simulink model "LoadPosition_simul"  (R2017a)
settings: Solver=FixedStepAuto  StartTime=0.0  StopTime=sim_time  FixedStep=delta  RelTol=1e-3
values from neighbouring files (symbols this model uses):
  A = [0.717 -1.367 -0.218 -0.867 -0.899 ... (first row only)    [LoadPosition_main.m]
  B = [0.083; 0.056; -0.056; 0.111; -0.056]    [LoadPosition_main.m]
  C = [0 1 1 0 0]    [LoadPosition_main.m]
  delta = 0.001    [LoadPosition_main.m]
  Dis_instant = 10    [LoadPosition_main.m]
  Dis_interval = 3    [LoadPosition_main.m]
  Dis_size = 5    [LoadPosition_main.m]
  K = place(A,B,poles)    [LoadPosition_main.m]
undefined symbols (not defined in the file or in its folder): A_, B_
settings Model: Creator=sihoon  LastModifiedBy=root

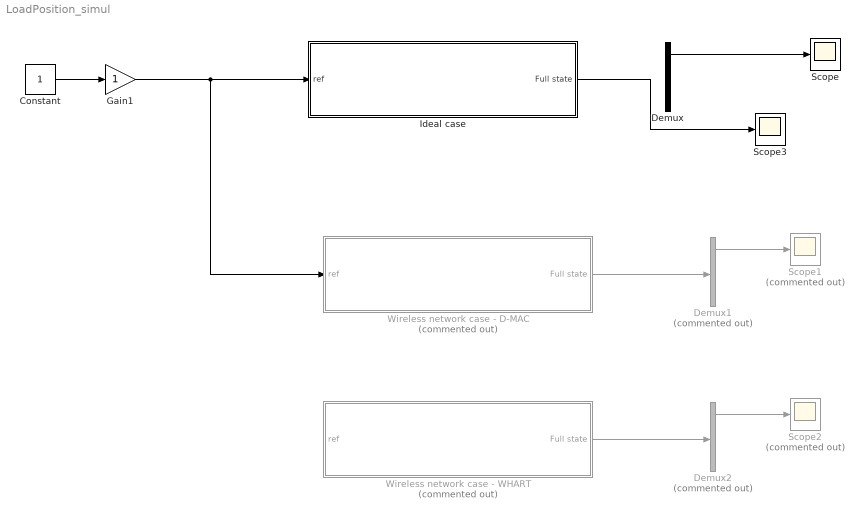
== system LoadPosition_simul ==
  Constant : Constant
  Demux : Demux
  Demux1 : Demux  Commented=on
  Demux2 : Demux  Commented=on
  Gain1 : Gain
  "Ideal case " : Subsystem
  Scope : Scope
  Scope1 : Scope  Commented=on
  Scope2 : Scope  Commented=on
  Scope3 : Scope
  Wireless network case - D-MAC : Subsystem  Commented=on
  Wireless network case - WHART : Subsystem  Commented=on
  wires:
  Constant/1 -> Gain1/1
  Demux/1 -> Scope/1
  "Ideal case "/1(Full state) -> Scope3/1
  Gain1/1 -> Wireless network case - D-MAC/1(ref), "Ideal case "/1(ref)
  Demux1/1 -> Scope1/1
  Wireless network case - D-MAC/1(Full state) -> Demux1/1
  Wireless network case - WHART/1(Full state) -> Demux2/1
  Demux2/1 -> Scope2/1

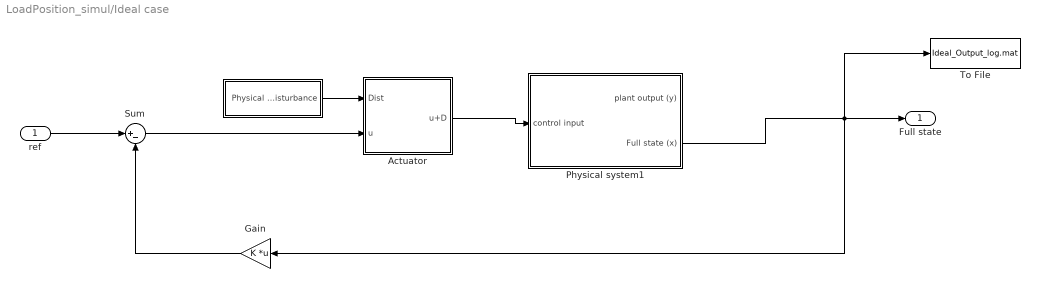
== system LoadPosition_simul/Ideal case  ==
  ref : Inport
  " " : Subsystem
  Actuator : Subsystem
  Gain : Gain  Gain=K  Multiplication=Matrix(K*u)
  Physical system1 : Subsystem
  Sum : Sum  Inputs=|+-
  To File : ToFile  Filename=Ideal_Output_log.mat  SaveFormat=Timeseries
  Full state : Outport
  wires:
  Physical system1/2(Full state (x)) -> Gain/1, Full state/1, To File/1
  Gain/1 -> Sum/2
  Sum/1 -> Actuator/2(u)
  ref/1 -> Sum/1
  " "/1(Physical Disturbance) -> Actuator/1(Dist)
  Actuator/1(u+D) -> Physical system1/1(control input)

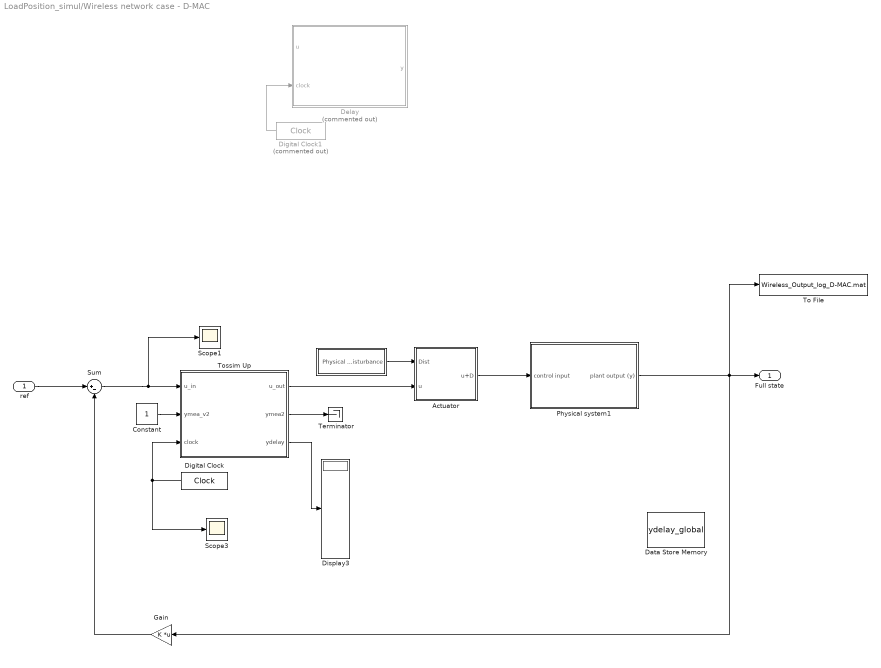
== system LoadPosition_simul/Wireless network case - D-MAC ==
  ref : Inport
  " " : Subsystem
  Actuator : Subsystem
  Constant : Constant
  Data Store Memory : DataStoreMemory  DataStoreName=ydelay_global  ReadBeforeWriteMsg=warning  WriteAfterWriteMsg=warning  WriteAfterReadMsg=warning  InitialValue=[1; 1; 1; 1; 1; 1; 1; 1; 1; 1; 1; 1; 1; 1; 1]  ShowAdditionalParam=off  OutDataTypeStr=uint32
  Delay : MATLAB Function  Commented=on  TreatAsAtomicUnit=on
  Digital Clock : DigitalClock  SampleTime=delta
  Digital Clock1 : DigitalClock  Commented=on  SampleTime=delta
  Display3 : Display
  Gain : Gain  Gain=K  Multiplication=Matrix(K*u)
  Physical system1 : Subsystem
  Scope1 : Scope
  Scope3 : Scope
  Sum : Sum  Inputs=|+-
  Terminator : Terminator
  To File : ToFile  Filename=Wireless_Output_log_D-MAC.mat  SaveFormat=Timeseries
  Tossim Up : MATLAB Function  TreatAsAtomicUnit=on
  Full state : Outport
  wires:
  Physical system1/1(plant output (y)) -> Gain/1, Full state/1, To File/1
  Gain/1 -> Sum/2
  ref/1 -> Sum/1
  Constant/1 -> Tossim Up/2(ymea_v2)
  Tossim Up/3(ydelay) -> Display3/1
  Digital Clock/1 -> Tossim Up/3(clock), Scope3/1
  Tossim Up/2(ymea2) -> Terminator/1
  Tossim Up/1(u_out) -> Actuator/2(u)
  Digital Clock1/1 -> Delay/2(clock)
  Sum/1 -> Tossim Up/1(u_in), Scope1/1
  " "/1(Physical Disturbance) -> Actuator/1(Dist)
  Actuator/1(u+D) -> Physical system1/1(control input)

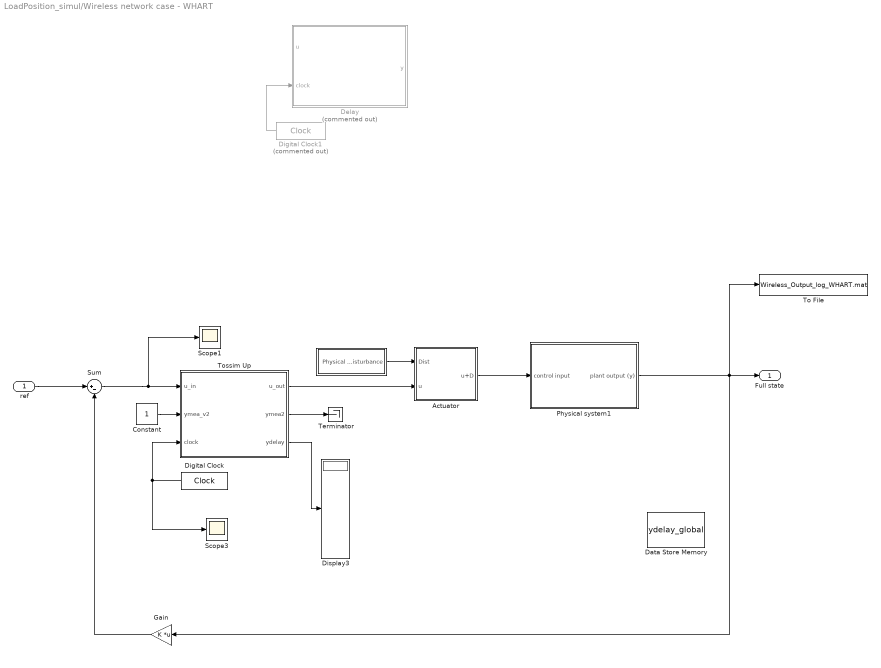
== system LoadPosition_simul/Wireless network case - WHART ==
  ref : Inport
  " " : Subsystem
  Actuator : Subsystem
  Constant : Constant
  Data Store Memory : DataStoreMemory  DataStoreName=ydelay_global  ReadBeforeWriteMsg=warning  WriteAfterWriteMsg=warning  WriteAfterReadMsg=warning  InitialValue=[1; 1; 1; 1; 1; 1; 1; 1; 1; 1; 1; 1; 1; 1; 1]  ShowAdditionalParam=off  OutDataTypeStr=uint32
  Delay : MATLAB Function  Commented=on  TreatAsAtomicUnit=on
  Digital Clock : DigitalClock  SampleTime=delta
  Digital Clock1 : DigitalClock  Commented=on  SampleTime=delta
  Display3 : Display
  Gain : Gain  Gain=K  Multiplication=Matrix(K*u)
  Physical system1 : Subsystem
  Scope1 : Scope
  Scope3 : Scope
  Sum : Sum  Inputs=|+-
  Terminator : Terminator
  To File : ToFile  Filename=Wireless_Output_log_WHART.mat  SaveFormat=Timeseries
  Tossim Up : MATLAB Function  TreatAsAtomicUnit=on
  Full state : Outport
  wires:
  Physical system1/1(plant output (y)) -> Gain/1, Full state/1, To File/1
  Gain/1 -> Sum/2
  ref/1 -> Sum/1
  Constant/1 -> Tossim Up/2(ymea_v2)
  Tossim Up/3(ydelay) -> Display3/1
  Digital Clock/1 -> Tossim Up/3(clock), Scope3/1
  Tossim Up/2(ymea2) -> Terminator/1
  Tossim Up/1(u_out) -> Actuator/2(u)
  Digital Clock1/1 -> Delay/2(clock)
  Sum/1 -> Tossim Up/1(u_in), Scope1/1
  " "/1(Physical Disturbance) -> Actuator/1(Dist)
  Actuator/1(u+D) -> Physical system1/1(control input)

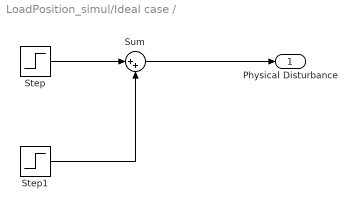
== system LoadPosition_simul/Ideal case /  ==
  Step : Step  Time=Dis_instant  After=Dis_size  SampleTime=0
  Step1 : Step  Time=Dis_instant+Dis_interval  After=-Dis_size  SampleTime=0
  Sum : Sum  Inputs=|++
  Physical Disturbance : Outport
  wires:
  Step/1 -> Sum/1
  Step1/1 -> Sum/2
  Sum/1 -> Physical Disturbance/1

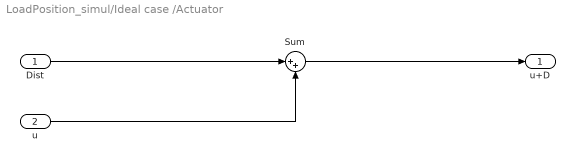
== system LoadPosition_simul/Ideal case /Actuator ==
  Dist : Inport
  u : Inport  Port=2
  Sum : Sum  Inputs=|++
  u+D : Outport
  wires:
  u/1 -> Sum/2
  Dist/1 -> Sum/1
  Sum/1 -> u+D/1

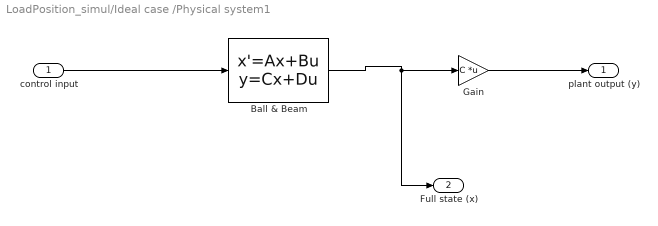
== system LoadPosition_simul/Ideal case /Physical system1 ==
  control input : Inport
  Ball & Beam : StateSpace  A=A  B=B  C=eye(5)  D=[0;0;0;0;0]  X0=0
  Gain : Gain  Gain=C  Multiplication=Matrix(K*u)
  plant output (y) : Outport
  Full state (x) : Outport  Port=2
  wires:
  control input/1 -> Ball & Beam/1
  Ball & Beam/1 -> Full state (x)/1, Gain/1
  Gain/1 -> plant output (y)/1

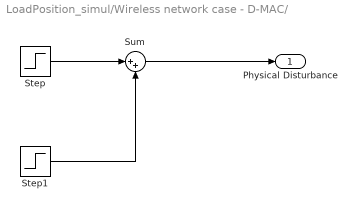
== system LoadPosition_simul/Wireless network case - D-MAC/  ==
  Step : Step  Time=Dis_instant  After=Dis_size  SampleTime=0
  Step1 : Step  Time=Dis_instant+Dis_interval  After=-Dis_size  SampleTime=0
  Sum : Sum  Inputs=|++
  Physical Disturbance : Outport
  wires:
  Step/1 -> Sum/1
  Step1/1 -> Sum/2
  Sum/1 -> Physical Disturbance/1

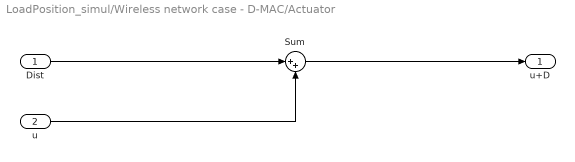
== system LoadPosition_simul/Wireless network case - D-MAC/Actuator ==
  Dist : Inport
  u : Inport  Port=2
  Sum : Sum  Inputs=|++
  u+D : Outport
  wires:
  u/1 -> Sum/2
  Dist/1 -> Sum/1
  Sum/1 -> u+D/1

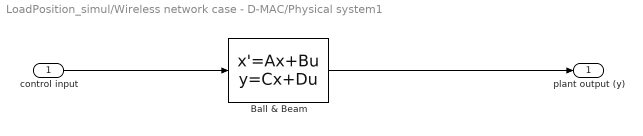
== system LoadPosition_simul/Wireless network case - D-MAC/Physical system1 ==
  control input : Inport
  Ball & Beam : StateSpace  A=A_  B=B_  C=eye(4)  D=[0;0;0;0]  X0=0
  plant output (y) : Outport
  wires:
  control input/1 -> Ball & Beam/1
  Ball & Beam/1 -> plant output (y)/1

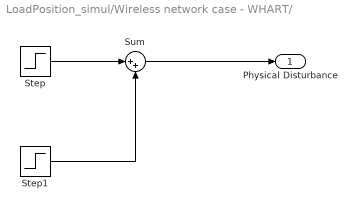
== system LoadPosition_simul/Wireless network case - WHART/  ==
  Step : Step  Time=Dis_instant  After=Dis_size  SampleTime=0
  Step1 : Step  Time=Dis_instant+Dis_interval  After=-Dis_size  SampleTime=0
  Sum : Sum  Inputs=|++
  Physical Disturbance : Outport
  wires:
  Step/1 -> Sum/1
  Step1/1 -> Sum/2
  Sum/1 -> Physical Disturbance/1

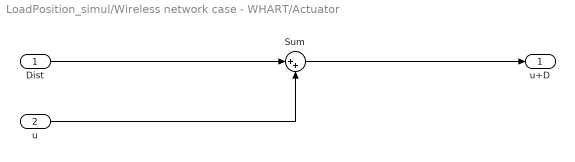
== system LoadPosition_simul/Wireless network case - WHART/Actuator ==
  Dist : Inport
  u : Inport  Port=2
  Sum : Sum  Inputs=|++
  u+D : Outport
  wires:
  u/1 -> Sum/2
  Dist/1 -> Sum/1
  Sum/1 -> u+D/1

== system LoadPosition_simul/Wireless network case - WHART/Physical system1 ==
  control input : Inport
  Ball & Beam : StateSpace  A=A  B=B  C=eye(4)  D=[0;0;0;0]  X0=0
  plant output (y) : Outport
  wires:
  control input/1 -> Ball & Beam/1
  Ball & Beam/1 -> plant output (y)/1

== matlab function LoadPosition_simul/Wireless network case - D-MAC/Tossim Up ==
  settings: updateMethod=DISCRETE
  data: u_out output; ymea2 output; u_in input; ydelay output; ydelay_global data_store_memory; ymea_v2 input; clock input
function [u_out,ymea2, ydelay]  = Tossim_block(u_in, ymea_v2, clock)
% Inputs:
% ymea: measurement from structure
% Outputs:
% ymea1: measurement output
% ydelay: delay traces
persistent past_u_in past_ymea_v2 % delay trace
persistent i Task_period % count 
persistent tossim_flag
global ydelay_global delta


% allow these matlab functions to be used in Embedded Matlab block
eml.extrinsic('python');
eml.extrinsic('num2str');
eml.extrinsic('str2num');
eml.extrinsic('delay_summary');
eml.extrinsic('disp');
eml.extrinsic('ps_aggregation');
eml.extrinsic('for');
eml.extrinsic('end');

if isempty(i)
    i = 0;
    %past_ymea = 0;
    past_u_in = u_in;
    past_ymea_v2 = ymea_v2;
    Task_period = [10 10 4];        %Task_period=[10 10 4] * 10
    tossim_flag = 0;
end

%[row column] = size(Task_period_time);

ydelay = [1 0 0 0 0 0 0 0 0]';
% call python to communicate with TOSSIM

% where clock increase with 1ms period
TOSSIM_step_size = 0.01;  % 10ms

call_count = 1; %Superframelength
rssi = -69;%sensor rssi

% Trigger Tossim once every 10ms
if mod(clock, TOSSIM_step_size) == 0
    if tossim_flag == 0
        tossim_flag = tossim_flag + 1;
        clock;
        [resultz] = ps_aggregation(call_count, rssi); %here call TOSSIM Client ----yh
        end_to_end_delivery_result_aggregated = sum(resultz);

        resultz;

        %[delay] = delay_summary(end_to_end_delivery_result_aggregated);
        [delay] = delay_summary(resultz);
        ydelay = delay';
    else
        resultz = [0 0 0 0 0 0 0 0];
        [delay] = delay_summary(resultz);
        ydelay = delay';
    end
else
    tossim_flag = 0;
    resultz = [0 0 0 0 0 0 0 0];
    [delay] = delay_summary(resultz);
    ydelay = delay';
end


% for event trigger!!!
% Packet arrive
%{
Task_period_time = Task_period * 10;
for j=Task_period_time(1,1:end)
    if(rem(clock,j) == 0)
        if(j == Task_period_time(1,1))      %Need to revise when # of Task is changed
           past_u_in = u_in;
        elseif(j == Task_period_time(1,2))
            past_ymea_v2 = ymea_v2;
        end
    end
end
%}

i = i+1;


for i_yg = 1:9
    ydelay_global(i_yg, 1) = ydelay(i_yg, 1);
end
delay = ydelay';

task1_index = 1;
ymea_v2_index = 2;
[delay_row delay_col] = size(delay);

for index = 1:delay_col
    
end
    
if delay(1,task1_index + 1)~=88
    u_out = past_u_in;
    past_u_in = u_in;
    %%%%
    ymea2 = past_ymea_v2;
elseif delay(1,ymea_v2_index + 1)~=88
    ymea2 = past_ymea_v2;
    past_ymea_v2 = ymea_v2;
    %%%
    u_out = past_u_in;
else
    u_out = past_u_in;
    ymea2 = past_ymea_v2;
end

== matlab function LoadPosition_simul/Wireless network case - D-MAC/Delay ==
  data: u input; y output; clock input
function y = fcn(u, clock)
persistent temp_clock prev_u i

if isempty(i)
    i=0;
    temp_clock = 0;
    prev_u = 0;
    
end

i = i+1;

% Transmission Period Test
Period = 0.1;


if mod(clock,Period) == 0
    y = prev_u;
    prev_u = u
    temp_clock = clock
else
    y = prev_u;
    
end
end

== matlab function LoadPosition_simul/Wireless network case - WHART/Delay ==
  data: u input; y output; clock input
function y = fcn(u, clock)
persistent temp_clock prev_u i

if isempty(i)
    i=0;
    temp_clock = 0;
    prev_u = 0;
    
end

i = i+1;

% Transmission Period Test
Period = 0.1;


if mod(clock,Period) == 0
    y = prev_u;
    prev_u = u
    temp_clock = clock
else
    y = prev_u;
    
end
end

== matlab function LoadPosition_simul/Wireless network case - WHART/Tossim Up ==
  settings: updateMethod=DISCRETE
  data: u_out output; ymea2 output; u_in input; ydelay output; ydelay_global data_store_memory; ymea_v2 input; clock input
function [u_out,ymea2, ydelay]  = Tossim_block(u_in, ymea_v2, clock)
% Inputs:
% ymea: measurement from structure
% Outputs:
% ymea1: measurement output
% ydelay: delay traces
persistent past_u_in past_ymea_v2 % delay trace
persistent i Task_period % count 
persistent tossim_flag
global ydelay_global delta


% allow these matlab functions to be used in Embedded Matlab block
eml.extrinsic('python');
eml.extrinsic('num2str');
eml.extrinsic('str2num');
eml.extrinsic('delay_summary');
eml.extrinsic('disp');
eml.extrinsic('ps_aggregation');
eml.extrinsic('for');
eml.extrinsic('end');

if isempty(i)
    i = 0;
    %past_ymea = 0;
    past_u_in = u_in;
    past_ymea_v2 = ymea_v2;
    Task_period = [10 10 4];        %Task_period=[10 10 4] * 10
    tossim_flag = 0;
end

%[row column] = size(Task_period_time);

ydelay = [1 0 0 0 0 0 0 0 0]';
% call python to communicate with TOSSIM

% where clock increase with 1ms period
TOSSIM_step_size = 0.01;  % 10ms

call_count = 1; %Superframelength
rssi = -69;%sensor rssi

% Trigger Tossim once every 10ms
if mod(clock, TOSSIM_step_size) == 0
    if tossim_flag == 0
        tossim_flag = tossim_flag + 1;
        clock;
        [resultz] = ps_aggregation(call_count, rssi); %here call TOSSIM Client ----yh
        end_to_end_delivery_result_aggregated = sum(resultz);

        resultz;

        %[delay] = delay_summary(end_to_end_delivery_result_aggregated);
        [delay] = delay_summary(resultz);
        ydelay = delay';
    else
        resultz = [0 0 0 0 0 0 0 0];
        [delay] = delay_summary(resultz);
        ydelay = delay';
    end
else
    tossim_flag = 0;
    resultz = [0 0 0 0 0 0 0 0];
    [delay] = delay_summary(resultz);
    ydelay = delay';
end


% for event trigger!!!
% Packet arrive
%{
Task_period_time = Task_period * 10;
for j=Task_period_time(1,1:end)
    if(rem(clock,j) == 0)
        if(j == Task_period_time(1,1))      %Need to revise when # of Task is changed
           past_u_in = u_in;
        elseif(j == Task_period_time(1,2))
            past_ymea_v2 = ymea_v2;
        end
    end
end
%}

i = i+1;


for i_yg = 1:9
    ydelay_global(i_yg, 1) = ydelay(i_yg, 1);
end
delay = ydelay';

task1_index = 1;
ymea_v2_index = 2;
[delay_row delay_col] = size(delay);

for index = 1:delay_col
    
end
    
if delay(1,task1_index + 1)~=88
    u_out = past_u_in;
    past_u_in = u_in;
    %%%%
    ymea2 = past_ymea_v2;
elseif delay(1,ymea_v2_index + 1)~=88
    ymea2 = past_ymea_v2;
    past_ymea_v2 = ymea_v2;
    %%%
    u_out = past_u_in;
else
    u_out = past_u_in;
    ymea2 = past_ymea_v2;
end
